simulink model "Simulation"  (R2024a)
settings: Solver=VariableStepAuto  StartTime=0.0  StopTime=10.0  RelTol=1e-3
values from neighbouring files (symbols this model uses):
  Ax = 0.3    [StateSpace.m]    (also in StateSpace00.m)
  Ay = 0.2    [StateSpace.m]    (also in StateSpace00.m)
  Az = 0.1    [StateSpace.m]    (also in StateSpace00.m)
  Cd = 0.4    [StateSpace.m]    (also in StateSpace00.m)
  g = 9.81    [StateSpace.m]    (also in StateSpace00.m = 9.8)
  Ix = (1/12) * m * (b^2 + c^2)    (= 0.416666666667)    [StateSpace.m]    (also in StateSpace00.m = 10)
  Iy = (1/12) * m * (a^2 + c^2)    (= 0.683333333333)    [StateSpace.m]    (also in StateSpace00.m = 20)
  Iz = (1/12) * m * (a^2 + b^2)    (= 0.566666666667)    [StateSpace.m]    (also in StateSpace00.m = 30)
  m = 5    [StateSpace.m]    (also in StateSpace00.m)
  rho = 1.225    [StateSpace.m]    (also in StateSpace00.m)
  T = 60    [StateSpace.m]    (also in StateSpace00.m = sqrt((Xp - 0)^2 + (Yp - 0)^2 + (Zp + 1)^2) * m * g)
  theta1 = 0.5    [StateSpace00.m]
  theta2 = 0.6    [StateSpace00.m]
settings Model: Creator=mscrobotic2324laptop1  LastModifiedBy=swh

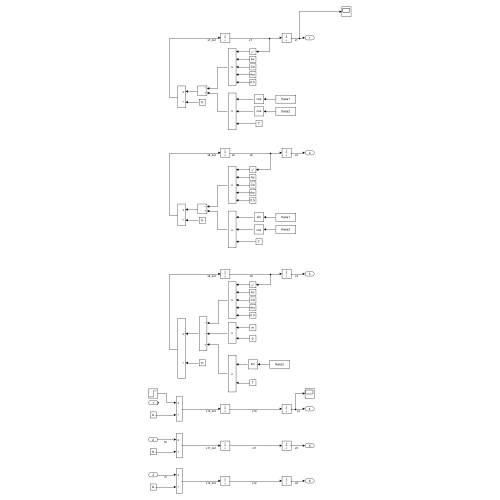
[thumbnail: Simulink's stored preview of the top-level diagram]
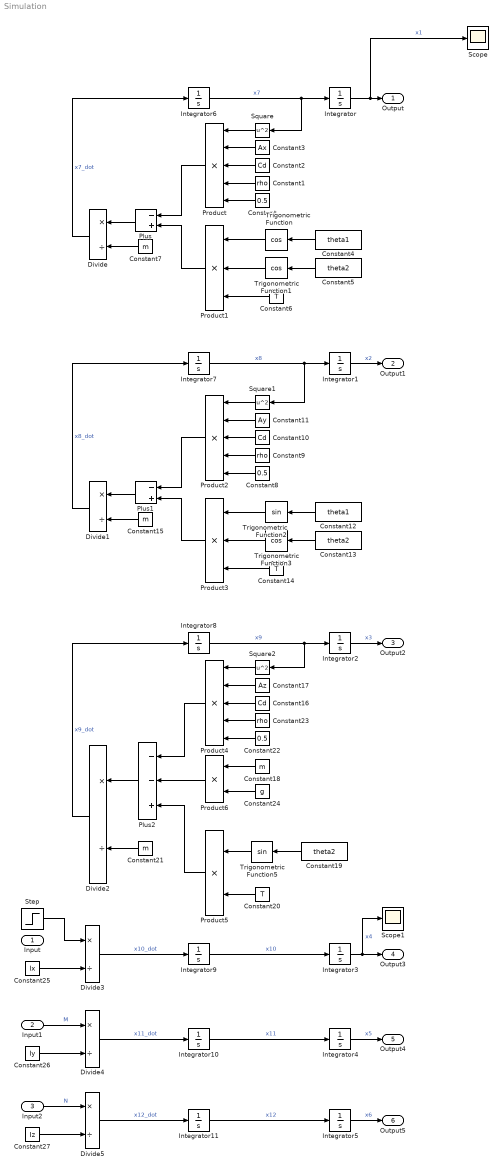
== system Simulation ==
  Input : Inport
  Input1 : Inport  Port=2
  Input2 : Inport  Port=3
  Constant : Constant  Value=0.5
  Constant1 : Constant  Value=rho
  Constant10 : Constant  Value=Cd
  Constant11 : Constant  Value=Ay
  Constant12 : Constant  Value=theta1
  Constant13 : Constant  Value=theta2
  Constant14 : Constant  Value=T
  Constant{7,15,18,21} (4 alike) : Constant  Value=m
  Constant16 : Constant  Value=Cd
  Constant17 : Constant  Value=Az
  Constant19 : Constant  Value=theta2
  Constant2 : Constant  Value=Cd
  Constant20 : Constant  Value=T
  Constant22 : Constant  Value=0.5
  Constant23 : Constant  Value=rho
  Constant24 : Constant  Value=g
  Constant25 : Constant  Value=Ix
  Constant26 : Constant  Value=Iy
  Constant27 : Constant  Value=Iz
  Constant3 : Constant  Value=Ax
  Constant4 : Constant  Value=theta1
  Constant5 : Constant  Value=theta2
  Constant6 : Constant  Value=T
  Constant8 : Constant  Value=0.5
  Constant9 : Constant  Value=rho
  Divide{,1..5} (6 alike) : Product  Inputs=*/
  Integrator{,1..11} (12 alike) : Integrator
  Plus : Sum  Inputs=-+
  Plus1 : Sum  Inputs=-+
  Plus2 : Sum  Inputs=--+
  Product : Product  Inputs=5
  Product1 : Product  Inputs=3
  Product2 : Product  Inputs=5
  Product3 : Product  Inputs=3
  Product4 : Product  Inputs=5
  Product5 : Product
  Product6 : Product
  Scope : Scope
  Scope1 : Scope
  Square : Math  Operator=square
  Square1 : Math  Operator=square
  Square2 : Math  Operator=square
  Step : Step  SampleTime=0
  Trigonometric Function : Trigonometry  Operator=cos
  Trigonometric Function1 : Trigonometry  Operator=cos
  Trigonometric Function2 : Trigonometry
  Trigonometric Function3 : Trigonometry  Operator=cos
  Trigonometric Function5 : Trigonometry
  Output : Outport
  Output1 : Outport  Port=2
  Output2 : Outport  Port=3
  Output3 : Outport  Port=4
  Output4 : Outport  Port=5
  Output5 : Outport  Port=6
  wires:
  Integrator6/1 -> Square/1, Integrator/1  "x7"
  Divide/1 -> Integrator6/1  "x7_dot"
  Divide1/1 -> Integrator7/1  "x8_dot"
  Divide2/1 -> Integrator8/1  "x9_dot"
  Divide3/1 -> Integrator9/1  "x10_dot"
  Divide4/1 -> Integrator10/1  "x11_dot"
  Divide5/1 -> Integrator11/1  "x12_dot"
  Integrator/1 -> Scope/1, Output/1  "x1"
  Integrator1/1 -> Output1/1  "x2"
  Integrator2/1 -> Output2/1  "x3"
  Integrator11/1 -> Integrator5/1  "x12"
  Integrator10/1 -> Integrator4/1  "x11"
  Integrator9/1 -> Integrator3/1  "x10"
  Integrator8/1 -> Square2/1, Integrator2/1  "x9"
  Integrator7/1 -> Square1/1, Integrator1/1  "x8"
  Integrator5/1 -> Output5/1  "x6"
  Integrator4/1 -> Output4/1  "x5"
  Integrator3/1 -> Scope1/1, Output3/1  "x4"
  Constant/1 -> Product/5
  Constant1/1 -> Product/4
  Square/1 -> Product/1
  Constant3/1 -> Product/2
  Constant2/1 -> Product/3
  Trigonometric Function/1 -> Product1/1
  Constant4/1 -> Trigonometric Function/1
  Constant5/1 -> Trigonometric Function1/1
  Trigonometric Function1/1 -> Product1/2
  Constant6/1 -> Product1/3
  Product/1 -> Plus/1
  Product1/1 -> Plus/2
  Plus/1 -> Divide/1
  Constant7/1 -> Divide/2
  Constant15/1 -> Divide1/2
  Trigonometric Function3/1 -> Product3/2
  Product2/1 -> Plus1/1
  Product3/1 -> Plus1/2
  Constant10/1 -> Product2/3
  Constant14/1 -> Product3/3
  Plus1/1 -> Divide1/1
  Constant12/1 -> Trigonometric Function2/1
  Constant13/1 -> Trigonometric Function3/1
  Constant9/1 -> Product2/4
  Trigonometric Function2/1 -> Product3/1
  Constant8/1 -> Product2/5
  Constant11/1 -> Product2/2
  Square1/1 -> Product2/1
  Constant17/1 -> Product4/2
  Constant22/1 -> Product4/5
  Constant20/1 -> Product5/2
  Constant16/1 -> Product4/3
  Constant21/1 -> Divide2/2
  Plus2/1 -> Divide2/1
  Constant19/1 -> Trigonometric Function5/1
  Product4/1 -> Plus2/1
  Constant23/1 -> Product4/4
  Square2/1 -> Product4/1
  Trigonometric Function5/1 -> Product5/1
  Product5/1 -> Plus2/3
  Constant18/1 -> Product6/1
  Constant24/1 -> Product6/2
  Product6/1 -> Plus2/2
  Constant25/1 -> Divide3/2
  Input1/1 -> Divide4/1  "M"
  Constant26/1 -> Divide4/2
  Input2/1 -> Divide5/1  "N"
  Constant27/1 -> Divide5/2
  Step/1 -> Divide3/1
